simulink model "matlabFun"  (R2020a)
settings: Solver=VariableStepAuto  StartTime=0.0  StopTime=10.0  RelTol=1e-3
settings Model: OrderedModelArguments=off  Creator=khoi  LastModifiedBy=khoi

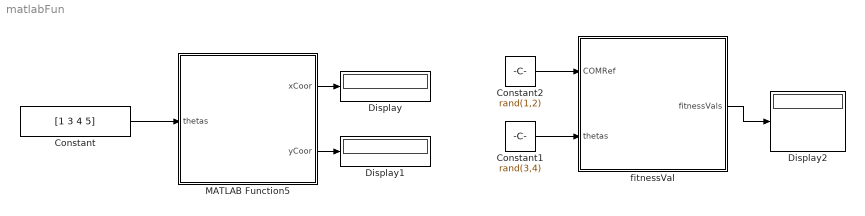
== system matlabFun ==
  Constant : Constant  Value=[1 3 4 5]
  Constant1 : Constant  Value=rand(3,4)
  Constant2 : Constant  Value=rand(1,2)
  Display : Display
  Display1 : Display
  Display2 : Display
  MATLAB Function5 : MATLAB Function  TreatAsAtomicUnit=on  mask{Len1=30, h1=10, Len2=400, Len3=500, l1=15, l2=200, l3=250, l4=300, m1=1, m2=5, m3=6, m4=10}
      mask prompts: Len1 "Feet (mm)"; h1 "Feet offset height (mm)"; Len2 "Lower leg (mm)"; Len3 "Upper leg (mm)"; l1 "Feet (mm)"; l2 "Lower leg (mm)"; l3 "Upper leg (mm)"; l4 "Upper body (mm)"; m1 "Feet (kg)"; m2 "Lower leg (kg)"; m3 "Upper leg (kg)"; m4 "Upper body (kg)"
  fitnessVal : MATLAB Function  TreatAsAtomicUnit=on  mask{Len1=30, h1=10, Len2=400, Len3=500, l1=15, l2=200, l3=250, l4=300, m1=1, m2=5, m3=6, m4=10}
      mask prompts: Len1 "Feet (mm)"; h1 "Feet offset height (mm)"; Len2 "Lower leg (mm)"; Len3 "Upper leg (mm)"; l1 "Feet (mm)"; l2 "Lower leg (mm)"; l3 "Upper leg (mm)"; l4 "Upper body (mm)"; m1 "Feet (kg)"; m2 "Lower leg (kg)"; m3 "Upper leg (kg)"; m4 "Upper body (kg)"
  wires:
  Constant/1 -> MATLAB Function5/1(thetas)
  MATLAB Function5/1(xCoor) -> Display/1
  MATLAB Function5/2(yCoor) -> Display1/1
  fitnessVal/1(fitnessVals) -> Display2/1
  Constant1/1 -> fitnessVal/2(thetas)
  Constant2/1 -> fitnessVal/1(COMRef)

== matlab function matlabFun/MATLAB Function5 ==
  data: h1 parameter; l1 parameter; l2 parameter; l3 parameter; l4 parameter; m1 parameter; m2 parameter; m3 parameter; m4 parameter; thetas input; xCoor output; yCoor output; Len1 parameter; Len2 parameter; Len3 parameter
function [xCoor,yCoor] = evalCOMTraj(h1,...
                           l1,l2,l3,l4,...
                           m1,m2,m3,m4,thetas, Len1, Len2, Len3)
    COM_est = COMTrajectory(Len1,Len2,Len3,h1,...
                           l1,l2,l3,l4,...
                           m1,m2,m3,m4,...
                           thetas(1),thetas(2),thetas(3),thetas(4));
    xCoor = COM_est(1);
    yCoor = COM_est(2);
end

== matlab function matlabFun/fitnessVal ==
  data: COMRef input; h1 parameter; l1 parameter; l2 parameter; l3 parameter; l4 parameter; m1 parameter; m2 parameter; m3 parameter; m4 parameter; Len1 parameter; Len2 parameter; Len3 parameter; thetas input; fitnessVals output
function fitnessVals = fitnessEval(COMRef, h1,...
                           l1,l2,l3,l4,...
                           m1,m2,m3,m4,...
                           Len1,Len2, Len3,...
                           thetas)
    COM_est = COMTrajectory(Len1,Len2,Len3,h1,...
                           l1,l2,l3,l4,...
                           m1,m2,m3,m4,...
                           thetas(:,1),thetas(:,2),thetas(:,3),thetas(:,4));
    COMRefMat = repmat(COMRef',size(COM_est,1),1);
    y = 1./(2*sqrt(dot(COM_est-COMRefMat,COM_est-COMRefMat,2)) + 1);
    fitnessVals = y;
end
